simulink library "InverterLIB"  (R2019a)
settings: Solver=VariableStepAuto  StartTime=0.0  StopTime=10.0  RelTol=1e-3
undefined symbols (not defined in the file or in its folder): fsw, Pmax, PolePairs, Tmax, Ts, Tsc, Vnom
libraries: fl_lib x17, nesl_utility x16, ee_lib x10, eePmsmFieldOrientedControl x2
settings Model: Creator=plewi  LastModifiedBy=plewi

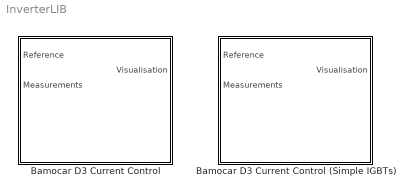
== system InverterLIB ==
  Bamocar D3 Current Control : Subsystem  mask(Bamocar D3){Vnom=Vnom, Pmax=Pmax, Tmax=Tmax, Iq_max=80, p=PolePairs, Vdc_on=10, Ts=2e-6, Tsc=5e-5, c=320, c_unit=uF, Vf=1.45, Ron=1e-3, Goff=1e-5, Vth=0.5, diode_Vf=1.55, diode_Ron=0.001, diode_Goff=1e-5, RefType=Zero d-axis control, psim=0.04, AxisAlignment=Q-axis, Kp_id=0.6, Ki_id=6, Kaw_id=100, Kp_iq=0.2, Ki_iq=8, Kaw_iq=100, AxisPrio=Q-axis, CPWMMode=SVM: space vector modulation, SamplingMode=Natural, fsw=2e3}
      mask prompts: Vnom "Nominal dc-link voltage (V):"; Pmax "Maximum power (W):"; Tmax "Maximum torque (N*m):"; Iq_max "Maximum current, Iq (A):"; p "Number of rotor pole pairs:"; Vdc_on "Inverter dc-link voltage threshold (V):"; Ts "Fundamental sample time (s):"; Tsc "Control sample time (s):"; c "Bank Capacitance"; Vf "Forward voltage, Vf (V):"; Ron "On-state resistance (Ohm):"; Goff "Off-state conductance (Siemens):"; Vth "Threshold voltage, Vth (V):"; diode_Vf "Forward voltage (V):"; diode_Ron "On resistance (Ohm):"; diode_Goff "Off conductance (Siemens):"; RefType "Current references:"; psim "Permanent magnet flux linkage (Wb):"; AxisAlignment "Phase-a axis alignment:"; Kp_id "D-axis current proportional gain:"; Ki_id "D-axis current integral gain:"; Kaw_id "D-axis current anti-windup gain:"; Kp_iq "Q-axis current proportional gain:"; Ki_iq "Q-axis current integral gain:"; Kaw_iq "Q-axis current anti-windup gain:"; AxisPrio "Axis prioritization:"; CPWMMode "PWM method:"; SamplingMode "Sampling mode:"; fsw "Switching frequency (Hz):"
      mask help: This block implements a PMSM field-oriented control structure, similar to the Bamocar D3. It operates under current/torque control.
      mask Help: web(nesl_help(gcbh))
      mask TypeOptions Vnom:
      | Inverter Controller/PMSM Field-Oriented
      | Control/Vnom
      mask TypeOptions Pmax:
      | Inverter Controller/PMSM Field-Oriented
      | Control/Pmax
      mask TypeOptions Tmax:
      | Inverter Controller/PMSM Field-Oriented
      | Control/Tmax
      mask TypeOptions p:
      | Inverter Controller/PMSM Field-Oriented
      | Control/p
      mask TypeOptions Vdc_on:
      | Inverter Controller/PMSM Field-Oriented
      | Control/Vdc_on
      mask TypeOptions Ts:
      | Inverter Controller/PMSM Field-Oriented
      | Control/Ts
      mask TypeOptions Tsc:
      | Inverter Controller/PMSM Field-Oriented
      | Control/Tsc
      mask TypeOptions c:
      | Three-Phase
      | Inverter/Capacitor
      | Bank/c
      mask TypeOptions c_unit:
      | Three-Phase
      | Inverter/Capacitor
      | Bank/c_unit
      mask TypeOptions Vf:
      | Three-Phase
      | Inverter/IGBT A(H)/Vf | Three-Phase
      | Inverter/IGBT A(L)/Vf | Three-Phase
      | Inverter/IGBT B(H)/Vf | Three-Phase
      | Inverter/IGBT B(L)/Vf | Three-Phase
      | Inverter/IGBT C(H)/Vf | Three-Phase
      | Inverter/IGBT C(L)/Vf
      mask TypeOptions Ron:
      | Three-Phase
      | Inverter/IGBT A(H)/Ron | Three-Phase
      | Inverter/IGBT A(L)/Ron | Three-Phase
      | Inverter/IGBT B(H)/Ron | Three-Phase
      | Inverter/IGBT B(L)/Ron | Three-Phase
      | Inverter/IGBT C(H)/Ron | Three-Phase
      | Inverter/IGBT C(L)/Ron
      mask TypeOptions Goff:
      | Three-Phase
      | Inverter/IGBT A(H)/Goff | Three-Phase
      | Inverter/IGBT A(L)/Goff | Three-Phase
      | Inverter/IGBT B(H)/Goff | Three-Phase
      | Inverter/IGBT B(L)/Goff | Three-Phase
      | Inverter/IGBT C(H)/Goff | Three-Phase
      | Inverter/IGBT C(L)/Goff
      mask TypeOptions Vth:
      | Three-Phase
      | Inverter/IGBT A(H)/Vth | Three-Phase
      | Inverter/IGBT A(L)/Vth | Three-Phase
      | Inverter/IGBT B(H)/Vth | Three-Phase
      | Inverter/IGBT B(L)/Vth | Three-Phase
      | Inverter/IGBT C(H)/Vth | Three-Phase
      | Inverter/IGBT C(L)/Vth
      mask TypeOptions diode_Vf:
      | Three-Phase
      | Inverter/IGBT A(H)/diode_Vf | Three-Phase
      | Inverter/IGBT A(L)/diode_Vf | Three-Phase
      | Inverter/IGBT B(H)/diode_Vf | Three-Phase
      | Inverter/IGBT B(L)/diode_Vf | Three-Phase
      | Inverter/IGBT C(H)/diode_Vf | Three-Phase
      | Inverter/IGBT C(L)/diode_Vf
      mask TypeOptions diode_Ron:
      | Three-Phase
      | Inverter/IGBT A(H)/diode_Ron | Three-Phase
      | Inverter/IGBT A(L)/diode_Ron | Three-Phase
      | Inverter/IGBT B(H)/diode_Ron | Three-Phase
      | Inverter/IGBT B(L)/diode_Ron | Three-Phase
      | Inverter/IGBT C(H)/diode_Ron | Three-Phase
      | Inverter/IGBT C(L)/diode_Ron
      mask TypeOptions diode_Goff:
      | Three-Phase
      | Inverter/IGBT A(H)/diode_Goff | Three-Phase
      | Inverter/IGBT A(L)/diode_Goff | Three-Phase
      | Inverter/IGBT B(H)/diode_Goff | Three-Phase
      | Inverter/IGBT B(L)/diode_Goff | Three-Phase
      | Inverter/IGBT C(H)/diode_Goff | Three-Phase
      | Inverter/IGBT C(L)/diode_Goff
      mask TypeOptions RefType:
      | Inverter Controller/PMSM Field-Oriented
      | Control/RefType
      mask TypeOptions psim:
      | Inverter Controller/PMSM Field-Oriented
      | Control/psim
      mask TypeOptions AxisAlignment:
      | Inverter Controller/PMSM Field-Oriented
      | Control/AxisAlignment
      mask TypeOptions Kp_id:
      | Inverter Controller/PMSM Field-Oriented
      | Control/Kp_id
      mask TypeOptions Ki_id:
      | Inverter Controller/PMSM Field-Oriented
      | Control/Ki_id
      mask TypeOptions Kaw_id:
      | Inverter Controller/PMSM Field-Oriented
      | Control/Kaw_id
      mask TypeOptions Kp_iq:
      | Inverter Controller/PMSM Field-Oriented
      | Control/Kp_iq
      mask TypeOptions Ki_iq:
      | Inverter Controller/PMSM Field-Oriented
      | Control/Ki_iq
      mask TypeOptions Kaw_iq:
      | Inverter Controller/PMSM Field-Oriented
      | Control/Kaw_iq
      mask TypeOptions AxisPrio:
      | Inverter Controller/PMSM Field-Oriented
      | Control/AxisPrio
      mask TypeOptions CPWMMode:
      | Inverter Controller/PMSM Field-Oriented
      | Control/CPWMMode
      mask TypeOptions SamplingMode:
      | Inverter Controller/PMSM Field-Oriented
      | Control/SamplingMode
      mask TypeOptions fsw:
      | Inverter Controller/PMSM Field-Oriented
      | Control/fsw
      mask DialogControl Container4 Prompt: General
      mask DialogControl Container11 Prompt: Electrical
      mask DialogControl Container12 Prompt: Capacitor Bank
      mask DialogControl Container16 Prompt: IGBTs
      mask DialogControl Container17 Prompt: Protection Diodes
      mask DialogControl Container5 Prompt: Outer Loop
      mask DialogControl Container6 Prompt: Inner Loop
      mask DialogControl Container7 Prompt: PWM
      mask Display: image('C:\Users\plewi\Documents\University\6-Sixth Year\MUR\MUR-E_Simulation_2019\Images\bamocar_d3.PNG');
  Bamocar D3 Current Control (Simple IGBTs) : Subsystem  mask(Bamocar D3 Current Controlled (Simple Diode)){Vnom=Vnom, Pmax=Pmax, Tmax=Tmax, Iq_max=80, p=PolePairs, Vdc_on=10, Ts=Ts, Tsc=Tsc, Ron=0.01, Goff=1e-8, Vf=0, diode_Vf=1.55, diode_Ron=0.01, diode_Goff=1e-8, RefType=Zero d-axis control, psim=0.04, AxisAlignment=Q-axis, Kp_id=0.6, Ki_id=6, Kaw_id=100, Kp_iq=0.2, Ki_iq=8, Kaw_iq=100, AxisPrio=Q-axis, CPWMMode=SVM: space vector modulation, SamplingMode=Natural, fsw=fsw}
      mask prompts: Vnom "Nominal dc-link voltage (V):"; Pmax "Maximum power (W):"; Tmax "Maximum torque (N*m):"; Iq_max "Maximum current, Iq (A):"; p "Number of rotor pole pairs:"; Vdc_on "Inverter dc-link voltage threshold (V):"; Ts "Fundamental sample time (s):"; Tsc "Control sample time (s):"; Ron "On-state resistance (Ohm):"; Goff "Off-state conductance (Siemens):"; Vf "Switching Threshold:"; diode_Vf "Forward voltage (V):"; diode_Ron "On resistance (Ohm):"; diode_Goff "Off conductance (Siemens):"; RefType "Current references:"; psim "Permanent magnet flux linkage (Wb):"; AxisAlignment "Phase-a axis alignment:"; Kp_id "D-axis current proportional gain:"; Ki_id "D-axis current integral gain:"; Kaw_id "D-axis current anti-windup gain:"; Kp_iq "Q-axis current proportional gain:"; Ki_iq "Q-axis current integral gain:"; Kaw_iq "Q-axis current anti-windup gain:"; AxisPrio "Axis prioritization:"; CPWMMode "PWM method:"; SamplingMode "Sampling mode:"; fsw "Switching frequency (Hz):"
      mask help: This block implements a PMSM field-oriented control structure, similar to the Bamocar D3. It operates under current/torque control.
      mask Help: web(nesl_help(gcbh))
      mask TypeOptions Vnom:
      | Inverter Controller/PMSM Field-Oriented
      | Control/Vnom
      mask TypeOptions Pmax:
      | Inverter Controller/PMSM Field-Oriented
      | Control/Pmax
      mask TypeOptions Tmax:
      | Inverter Controller/PMSM Field-Oriented
      | Control/Tmax
      mask TypeOptions p:
      | Inverter Controller/PMSM Field-Oriented
      | Control/p
      mask TypeOptions Vdc_on:
      | Inverter Controller/PMSM Field-Oriented
      | Control/Vdc_on
      mask TypeOptions Ts:
      | Inverter Controller/PMSM Field-Oriented
      | Control/Ts
      mask TypeOptions Tsc:
      | Inverter Controller/PMSM Field-Oriented
      | Control/Tsc
      mask TypeOptions Ron:
      | Three-Phase
      | Inverter/Switch/R_closed | Three-Phase
      | Inverter/Switch1/R_closed | Three-Phase
      | Inverter/Switch2/R_closed | Three-Phase
      | Inverter/Switch3/R_closed | Three-Phase
      | Inverter/Switch4/R_closed | Three-Phase
      | Inverter/Switch5/R_closed
      mask TypeOptions Goff:
      | Three-Phase
      | Inverter/Switch/G_open | Three-Phase
      | Inverter/Switch1/G_open | Three-Phase
      | Inverter/Switch2/G_open | Three-Phase
      | Inverter/Switch3/G_open | Three-Phase
      | Inverter/Switch4/G_open | Three-Phase
      | Inverter/Switch5/G_open
      mask TypeOptions Vf:
      | Three-Phase
      | Inverter/Switch/Threshold | Three-Phase
      | Inverter/Switch1/Threshold | Three-Phase
      | Inverter/Switch2/Threshold | Three-Phase
      | Inverter/Switch3/Threshold | Three-Phase
      | Inverter/Switch4/Threshold | Three-Phase
      | Inverter/Switch5/Threshold
      mask TypeOptions diode_Vf:
      | Three-Phase
      | Inverter/Diode1/Vf | Three-Phase
      | Inverter/Diode2/Vf | Three-Phase
      | Inverter/Diode3/Vf | Three-Phase
      | Inverter/Diode4/Vf | Three-Phase
      | Inverter/Diode5/Vf | Three-Phase
      | Inverter/Diode6/Vf
      mask TypeOptions diode_Ron:
      | Three-Phase
      | Inverter/Diode1/Ron | Three-Phase
      | Inverter/Diode2/Ron | Three-Phase
      | Inverter/Diode3/Ron | Three-Phase
      | Inverter/Diode4/Ron | Three-Phase
      | Inverter/Diode5/Ron | Three-Phase
      | Inverter/Diode6/Ron
      mask TypeOptions diode_Goff:
      | Three-Phase
      | Inverter/Diode1/Goff | Three-Phase
      | Inverter/Diode2/Goff | Three-Phase
      | Inverter/Diode3/Goff | Three-Phase
      | Inverter/Diode4/Goff | Three-Phase
      | Inverter/Diode5/Goff | Three-Phase
      | Inverter/Diode6/Goff
      mask TypeOptions RefType:
      | Inverter Controller/PMSM Field-Oriented
      | Control/RefType
      mask TypeOptions psim:
      | Inverter Controller/PMSM Field-Oriented
      | Control/psim
      mask TypeOptions AxisAlignment:
      | Inverter Controller/PMSM Field-Oriented
      | Control/AxisAlignment
      mask TypeOptions Kp_id:
      | Inverter Controller/PMSM Field-Oriented
      | Control/Kp_id
      mask TypeOptions Ki_id:
      | Inverter Controller/PMSM Field-Oriented
      | Control/Ki_id
      mask TypeOptions Kaw_id:
      | Inverter Controller/PMSM Field-Oriented
      | Control/Kaw_id
      mask TypeOptions Kp_iq:
      | Inverter Controller/PMSM Field-Oriented
      | Control/Kp_iq
      mask TypeOptions Ki_iq:
      | Inverter Controller/PMSM Field-Oriented
      | Control/Ki_iq
      mask TypeOptions Kaw_iq:
      | Inverter Controller/PMSM Field-Oriented
      | Control/Kaw_iq
      mask TypeOptions AxisPrio:
      | Inverter Controller/PMSM Field-Oriented
      | Control/AxisPrio
      mask TypeOptions CPWMMode:
      | Inverter Controller/PMSM Field-Oriented
      | Control/CPWMMode
      mask TypeOptions SamplingMode:
      | Inverter Controller/PMSM Field-Oriented
      | Control/SamplingMode
      mask TypeOptions fsw:
      | Inverter Controller/PMSM Field-Oriented
      | Control/fsw
      mask DialogControl Container4 Prompt: General
      mask DialogControl Container11 Prompt: Electrical
      mask DialogControl Container12 Prompt: Capacitor Bank
      mask DialogControl Container16 Prompt: IGBTs
      mask DialogControl Container17 Prompt: Protection Diodes
      mask DialogControl Container5 Prompt: Outer Loop
      mask DialogControl Container6 Prompt: Inner Loop
      mask DialogControl Container7 Prompt: PWM
      mask Display: image('C:\Users\plewi\Documents\University\6-Sixth Year\MUR\MUR-E_Simulation_2019\Images\bamocar_d3.PNG');

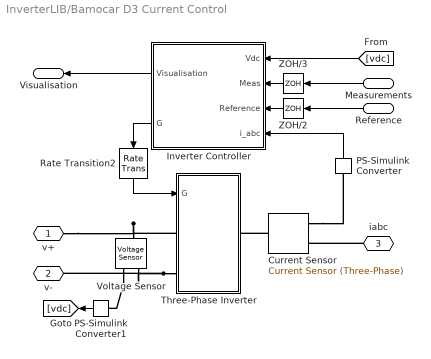
== system InverterLIB/Bamocar D3 Current Control ==
  Reference : Inport
  Measurements : Inport  Port=2
  Current Sensor : ee_lib/Sensors & Transducers/Current Sensor (Three-Phase)
      settings: SourceProductName=Simscape Electrical
  Inverter Controller : Subsystem
  PS-Simulink Converter : nesl_utility/PS-Simulink Converter  PhysicalDomain=network_engine_domain  SubClassName=ps_output  LeftPortType=input  RightPortType=output  PseudoPeriodic=off  Frequencies=[]  Unit=1  AffineConversion=off
  PS-Simulink Converter1 : nesl_utility/PS-Simulink Converter  PhysicalDomain=network_engine_domain  SubClassName=ps_output  LeftPortType=input  RightPortType=output  PseudoPeriodic=off  Frequencies=[]  Unit=1  AffineConversion=off
  Rate Transition2 : RateTransition  OutPortSampleTime=Ts
  Three-Phase Inverter : Subsystem
  Voltage Sensor : fl_lib/Electrical/Electrical Sensors/Voltage Sensor
  ZOH/2 : ZeroOrderHold  SampleTime=Tsc
  ZOH/3 : ZeroOrderHold  SampleTime=Tsc
  v+ : PMIOPort  Side=Left
  v- : PMIOPort  Port=2  Side=Left
  iabc : PMIOPort  Port=3  Side=Right
  Visualisation : Outport
  wires:
  PS-Simulink Converter/1 -> Inverter Controller/4(i_abc)
  ZOH/2/1 -> Inverter Controller/3(Reference)
  Rate Transition2/1 -> Three-Phase Inverter/1(G)
  Measurements/1 -> ZOH/3/1
  Inverter Controller/1(Visualisation) -> Visualisation/1
  PS-Simulink Converter1/1 -> [vdc]
  Inverter Controller/2(G) -> Rate Transition2/1
  [vdc] -> Inverter Controller/1(Vdc)
  ZOH/3/1 -> Inverter Controller/2(Meas)
  Reference/1 -> ZOH/2/1
  connections:
  Voltage Sensor/LConn1 -- v+/RConn1 -- Three-Phase Inverter/LConn1
  Three-Phase Inverter/LConn2 -- v-/RConn1 -- Voltage Sensor/RConn2
  Current Sensor/LConn1 -- Three-Phase Inverter/RConn1
  Current Sensor/RConn1 -- PS-Simulink Converter/LConn1
  Voltage Sensor/RConn1 -- PS-Simulink Converter1/LConn1
  iabc/RConn1 -- Current Sensor/RConn2

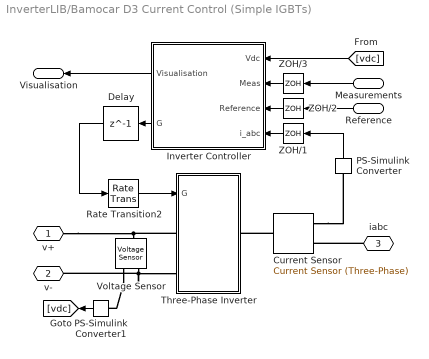
== system InverterLIB/Bamocar D3 Current Control (Simple IGBTs) ==
  Reference : Inport
  Measurements : Inport  Port=2
  Current Sensor : ee_lib/Sensors & Transducers/Current Sensor (Three-Phase)
      settings: SourceProductName=Simscape Electrical
  Delay : Delay  DelayLength=1
  Inverter Controller : Subsystem
  PS-Simulink Converter : nesl_utility/PS-Simulink Converter  PhysicalDomain=network_engine_domain  SubClassName=ps_output  LeftPortType=input  RightPortType=output  PseudoPeriodic=off  Frequencies=[]  Unit=1  AffineConversion=off
  PS-Simulink Converter1 : nesl_utility/PS-Simulink Converter  PhysicalDomain=network_engine_domain  SubClassName=ps_output  LeftPortType=input  RightPortType=output  PseudoPeriodic=off  Frequencies=[]  Unit=1  AffineConversion=off
  Rate Transition2 : RateTransition  OutPortSampleTime=Ts
  Three-Phase Inverter : Subsystem
  Voltage Sensor : fl_lib/Electrical/Electrical Sensors/Voltage Sensor
  ZOH/1 : ZeroOrderHold  SampleTime=Tsc
  ZOH/2 : ZeroOrderHold  SampleTime=Tsc
  ZOH/3 : ZeroOrderHold  SampleTime=Tsc
  v+ : PMIOPort  Side=Left
  v- : PMIOPort  Port=2  Side=Left
  iabc : PMIOPort  Port=3  Side=Right
  Visualisation : Outport
  wires:
  Reference/1 -> ZOH/2/1
  ZOH/3/1 -> Inverter Controller/2(Meas)
  [vdc] -> Inverter Controller/1(Vdc)
  PS-Simulink Converter1/1 -> [vdc]
  Inverter Controller/1(Visualisation) -> Visualisation/1
  Rate Transition2/1 -> Three-Phase Inverter/1(G)
  ZOH/2/1 -> Inverter Controller/3(Reference)
  PS-Simulink Converter/1 -> ZOH/1/1
  ZOH/1/1 -> Inverter Controller/4(i_abc)
  Inverter Controller/2(G) -> Delay/1
  Delay/1 -> Rate Transition2/1
  Measurements/1 -> ZOH/3/1
  connections:
  iabc/RConn1 -- Current Sensor/RConn2
  Voltage Sensor/RConn1 -- PS-Simulink Converter1/LConn1
  Current Sensor/RConn1 -- PS-Simulink Converter/LConn1
  Current Sensor/LConn1 -- Three-Phase Inverter/RConn1
  Voltage Sensor/RConn2 -- v-/RConn1 -- Three-Phase Inverter/LConn2
  Three-Phase Inverter/LConn1 -- v+/RConn1 -- Voltage Sensor/LConn1

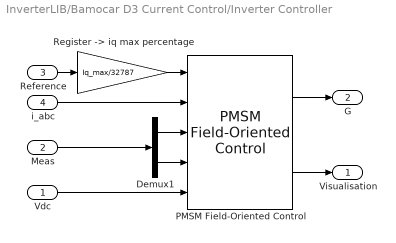
== system InverterLIB/Bamocar D3 Current Control/Inverter Controller ==
  Vdc : Inport
  Meas : Inport  Port=2
  Reference : Inport  Port=3
  i_abc : Inport  Port=4
  Demux1 : Demux  Outputs=2
  PMSM Field-Oriented Control : eePmsmFieldOrientedControl/PMSM Field-Oriented Control  CtrlMode=Torque control  Vnom=Vnom  Pmax=Pmax  Tmax=Tmax  p=p  Vdc_on=Vdc_on  Ts=Ts  Tsc=Tsc  CtrlType=PI control  Kp_w=50  Ki_w=500  Kv_w=1  Kaw_w=1000  RefType=Zero d-axis control  rpmVec=[0, 3000]  TqVec=[-100, 0, 100]  VdcVec=[300, 350]  idMatrix=zeros(2,3,2)  iqMatrix=zeros(2,3,2)  psim=psim  Ld=0.00024  Lq=0.00029  Rs=0.01  AxisAlignment=Q-axis  Kp_id=Kp_id  Ki_id=Ki_id  Kaw_id=Kaw_id  Kp_iq=Kp_iq  Ki_iq=Ki_iq  Kaw_iq=Kaw_iq  AxisPrio=Q-axis  ActZC=on  ActFF=off  ParamTypeFF=Constant parameters  LdFF=Ld  LqFF=Lq  psimFF=PM  idVect=[-200, 0, 200]  iqVect=[-200, 0, 200]  LdMatrix=0.0002 * ones(3, 3)  LqMatrix=0.0002 * ones(3, 3)  psimMatrix=0.04 * ones(3, 3)  CPWMMode=SVM: space vector modulation  fsw=fsw
      settings: SourceProductName=Simscape Electrical  SourceProductBaseCode=PS
  "Register -> iq max percentage" : Gain  Gain=Iq_max/32787
  Visualisation : Outport
  G : Outport  Port=2
  wires:
  PMSM Field-Oriented Control/1 -> G/1
  Vdc/1 -> PMSM Field-Oriented Control/5
  PMSM Field-Oriented Control/2 -> Visualisation/1
  i_abc/1 -> PMSM Field-Oriented Control/2
  Meas/1 -> Demux1/1
  Demux1/1 -> PMSM Field-Oriented Control/3
  Demux1/2 -> PMSM Field-Oriented Control/4
  "Register -> iq max percentage"/1 -> PMSM Field-Oriented Control/1
  Reference/1 -> "Register -> iq max percentage"/1

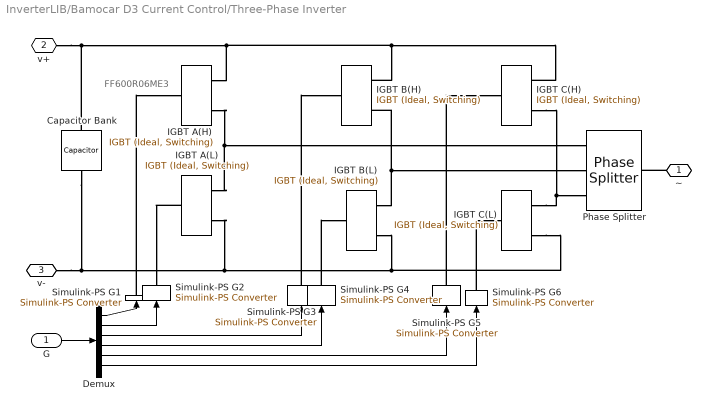
== system InverterLIB/Bamocar D3 Current Control/Three-Phase Inverter ==
  note: FF600R06ME3
  G : Inport
  Capacitor Bank : fl_lib/Electrical/Electrical Elements/Capacitor  c=c uF  r=0 Ohm  g=0 1/Ohm  i_specify=off  i_priority=None  i=0 A  i_nominal_specify=off  i_nominal_unit=A  i_nominal_value=1  v_specify=off  v_priority=None  v=0 V  v_nominal_specify=off  v_nominal_unit=V  v_nominal_value=1  vc_specify=off  vc_priority=High  vc=0 V  vc_nominal_specify=off  vc_nominal_unit=V  vc_nominal_value=1
  Demux : Demux  Outputs=6
  IGBT A(H) : ee_lib/Semiconductors & Converters/IGBT (Ideal, Switching)  Description=Bamocar D3 IGBT Model Number: FF600R06ME3  Vf=Vf V  Ron=Ron Ohm  Goff=Goff S  Vth=Vth V  diode_param=2  diode_Vf=diode_Vf V  diode_Ron=diode_Ron Ohm  diode_Goff=diode_Goff S  diode_C=5e-8 F  diode_iRM=-235 A  diode_iF=300 A  diode_idot=-50 A/us  diode_trr_param=1  diode_trr_factor=3  diode_trr=15 us  diode_Qrr=1.5e+3 s*uA  thermal_loss_option=2  Voff=300 V  Tau=1e-4 s  Tj=[298.15, 398.15] K  Iout_scalar=600 A  Eon_scalar=22.86e-3 J  Eoff_scalar=17.14e-3 J  Von_scalar=2.7 V  Iout_data=[0, 10, 50, 100, 200, 400, 600] A  Eon_data=[0, .29, 1.43, 2.86, 5.71, 13.14, 22.86; 0, .57, 2.63, 5.14, 10.29, 20.57, 30.29] * 1e-3 J  Eoff_data=[0, .21, 1.07, 2.14, 4.29, 9.86, 17.14; 0, .43, 1.97, 3.86, 7.71, 15.43, 22.71] * 1e-3 J  Von_data=[0, 1.1, 1.3, 1.45, 1.75, 2.25, 2.7; 0, 1, 1.15, 1.35, 1.7, 2.35, 3] V
      settings: SourceProductName=Simscape Electrical
  IGBT A(L) : ee_lib/Semiconductors & Converters/IGBT (Ideal, Switching)  Description=Bamocar D3 IGBT Model Number: FF600R06ME3  Vf=Vf V  Ron=Ron Ohm  Goff=Goff S  Vth=Vth V  diode_param=2  diode_Vf=diode_Vf V  diode_Ron=diode_Ron Ohm  diode_Goff=diode_Goff S  diode_C=5e-8 F  diode_iRM=-235 A  diode_iF=300 A  diode_idot=-50 A/us  diode_trr_param=1  diode_trr_factor=3  diode_trr=15 us  diode_Qrr=1.5e+3 s*uA  thermal_loss_option=2  Voff=300 V  Tau=1e-4 s  Tj=[298.15, 398.15] K  Iout_scalar=600 A  Eon_scalar=22.86e-3 J  Eoff_scalar=17.14e-3 J  Von_scalar=2.7 V  Iout_data=[0, 10, 50, 100, 200, 400, 600] A  Eon_data=[0, .29, 1.43, 2.86, 5.71, 13.14, 22.86; 0, .57, 2.63, 5.14, 10.29, 20.57, 30.29] * 1e-3 J  Eoff_data=[0, .21, 1.07, 2.14, 4.29, 9.86, 17.14; 0, .43, 1.97, 3.86, 7.71, 15.43, 22.71] * 1e-3 J  Von_data=[0, 1.1, 1.3, 1.45, 1.75, 2.25, 2.7; 0, 1, 1.15, 1.35, 1.7, 2.35, 3] V
      settings: SourceProductName=Simscape Electrical
  IGBT B(H) : ee_lib/Semiconductors & Converters/IGBT (Ideal, Switching)  Description=Bamocar D3 IGBT Model Number: FF600R06ME3  Vf=Vf V  Ron=Ron Ohm  Goff=Goff S  Vth=Vth V  diode_param=2  diode_Vf=diode_Vf V  diode_Ron=diode_Ron Ohm  diode_Goff=diode_Goff S  diode_C=5e-8 F  diode_iRM=-235 A  diode_iF=300 A  diode_idot=-50 A/us  diode_trr_param=1  diode_trr_factor=3  diode_trr=15 us  diode_Qrr=1.5e+3 s*uA  thermal_loss_option=2  Voff=300 V  Tau=1e-4 s  Tj=[298.15, 398.15] K  Iout_scalar=600 A  Eon_scalar=22.86e-3 J  Eoff_scalar=17.14e-3 J  Von_scalar=2.7 V  Iout_data=[0, 10, 50, 100, 200, 400, 600] A  Eon_data=[0, .29, 1.43, 2.86, 5.71, 13.14, 22.86; 0, .57, 2.63, 5.14, 10.29, 20.57, 30.29] * 1e-3 J  Eoff_data=[0, .21, 1.07, 2.14, 4.29, 9.86, 17.14; 0, .43, 1.97, 3.86, 7.71, 15.43, 22.71] * 1e-3 J  Von_data=[0, 1.1, 1.3, 1.45, 1.75, 2.25, 2.7; 0, 1, 1.15, 1.35, 1.7, 2.35, 3] V
      settings: SourceProductName=Simscape Electrical
  IGBT B(L) : ee_lib/Semiconductors & Converters/IGBT (Ideal, Switching)  Description=Bamocar D3 IGBT Model Number: FF600R06ME3  Vf=Vf V  Ron=Ron Ohm  Goff=Goff S  Vth=Vth V  diode_param=2  diode_Vf=diode_Vf V  diode_Ron=diode_Ron Ohm  diode_Goff=diode_Goff S  diode_C=5e-8 F  diode_iRM=-235 A  diode_iF=300 A  diode_idot=-50 A/us  diode_trr_param=1  diode_trr_factor=3  diode_trr=15 us  diode_Qrr=1.5e+3 s*uA  thermal_loss_option=2  Voff=300 V  Tau=1e-4 s  Tj=[298.15, 398.15] K  Iout_scalar=600 A  Eon_scalar=22.86e-3 J  Eoff_scalar=17.14e-3 J  Von_scalar=2.7 V  Iout_data=[0, 10, 50, 100, 200, 400, 600] A  Eon_data=[0, .29, 1.43, 2.86, 5.71, 13.14, 22.86; 0, .57, 2.63, 5.14, 10.29, 20.57, 30.29] * 1e-3 J  Eoff_data=[0, .21, 1.07, 2.14, 4.29, 9.86, 17.14; 0, .43, 1.97, 3.86, 7.71, 15.43, 22.71] * 1e-3 J  Von_data=[0, 1.1, 1.3, 1.45, 1.75, 2.25, 2.7; 0, 1, 1.15, 1.35, 1.7, 2.35, 3] V
      settings: SourceProductName=Simscape Electrical
  IGBT C(H) : ee_lib/Semiconductors & Converters/IGBT (Ideal, Switching)  Description=Bamocar D3 IGBT Model Number: FF600R06ME3  Vf=Vf V  Ron=Ron Ohm  Goff=Goff S  Vth=Vth V  diode_param=2  diode_Vf=diode_Vf V  diode_Ron=diode_Ron Ohm  diode_Goff=diode_Goff S  diode_C=5e-8 F  diode_iRM=-235 A  diode_iF=300 A  diode_idot=-50 A/us  diode_trr_param=1  diode_trr_factor=3  diode_trr=15 us  diode_Qrr=1.5e+3 s*uA  thermal_loss_option=2  Voff=300 V  Tau=1e-4 s  Tj=[298.15, 398.15] K  Iout_scalar=600 A  Eon_scalar=22.86e-3 J  Eoff_scalar=17.14e-3 J  Von_scalar=2.7 V  Iout_data=[0, 10, 50, 100, 200, 400, 600] A  Eon_data=[0, .29, 1.43, 2.86, 5.71, 13.14, 22.86; 0, .57, 2.63, 5.14, 10.29, 20.57, 30.29] * 1e-3 J  Eoff_data=[0, .21, 1.07, 2.14, 4.29, 9.86, 17.14; 0, .43, 1.97, 3.86, 7.71, 15.43, 22.71] * 1e-3 J  Von_data=[0, 1.1, 1.3, 1.45, 1.75, 2.25, 2.7; 0, 1, 1.15, 1.35, 1.7, 2.35, 3] V
      settings: SourceProductName=Simscape Electrical
  IGBT C(L) : ee_lib/Semiconductors & Converters/IGBT (Ideal, Switching)  Description=Bamocar D3 IGBT Model Number: FF600R06ME3  Vf=Vf V  Ron=Ron Ohm  Goff=Goff S  Vth=Vth V  diode_param=2  diode_Vf=diode_Vf V  diode_Ron=diode_Ron Ohm  diode_Goff=diode_Goff S  diode_C=5e-8 F  diode_iRM=-235 A  diode_iF=300 A  diode_idot=-50 A/us  diode_trr_param=1  diode_trr_factor=3  diode_trr=15 us  diode_Qrr=1.5e+3 s*uA  thermal_loss_option=2  Voff=300 V  Tau=1e-4 s  Tj=[298.15, 398.15] K  Iout_scalar=600 A  Eon_scalar=22.86e-3 J  Eoff_scalar=17.14e-3 J  Von_scalar=2.7 V  Iout_data=[0, 10, 50, 100, 200, 400, 600] A  Eon_data=[0, .29, 1.43, 2.86, 5.71, 13.14, 22.86; 0, .57, 2.63, 5.14, 10.29, 20.57, 30.29] * 1e-3 J  Eoff_data=[0, .21, 1.07, 2.14, 4.29, 9.86, 17.14; 0, .43, 1.97, 3.86, 7.71, 15.43, 22.71] * 1e-3 J  Von_data=[0, 1.1, 1.3, 1.45, 1.75, 2.25, 2.7; 0, 1, 1.15, 1.35, 1.7, 2.35, 3] V
      settings: SourceProductName=Simscape Electrical
  Phase Splitter : ee_lib/Connectors & References/Phase Splitter
      settings: SourceProductName=Simscape Electrical  SourceProductBaseCode=PS
  Simulink-PS G{1..6} (6 alike) : nesl_utility/Simulink-PS Converter  PhysicalDomain=network_engine_domain  SubClassName=ps_input  LeftPortType=input  RightPortType=output  PseudoPeriodic=off  Frequencies=[]  NoiseDistribution=none  NoiseParameters=[]  Unit=1  AffineConversion=off  FilteringAndDerivatives=zero  SimscapeFilterOrder=1  InputFilterTimeConstant=1e-6  UdotUserProvided=0
  ~ : PMIOPort  Tag=PMCPort  Side=Right
  v+ : PMIOPort  Tag=PMCPort  Port=2  Side=Left
  v- : PMIOPort  Tag=PMCPort  Port=3  Side=Left
  wires:
  Demux/5 -> Simulink-PS G5/1
  Demux/4 -> Simulink-PS G4/1
  Demux/3 -> Simulink-PS G3/1
  Demux/2 -> Simulink-PS G2/1
  Demux/1 -> Simulink-PS G1/1
  G/1 -> Demux/1
  Demux/6 -> Simulink-PS G6/1
  connections:
  Simulink-PS G6/RConn1 -- IGBT C(L)/LConn1
  Simulink-PS G5/RConn1 -- IGBT C(H)/LConn1
  Simulink-PS G4/RConn1 -- IGBT B(L)/LConn1
  Simulink-PS G3/RConn1 -- IGBT B(H)/LConn1
  IGBT B(L)/RConn2 -- v-/RConn1 -- Capacitor Bank/RConn1 -- IGBT A(L)/RConn2 -- IGBT C(L)/RConn2
  IGBT A(H)/RConn2 -- Phase Splitter/RConn1 -- IGBT A(L)/RConn1
  IGBT B(L)/RConn1 -- Phase Splitter/RConn2 -- IGBT B(H)/RConn2
  IGBT C(L)/RConn1 -- Phase Splitter/RConn3 -- IGBT C(H)/RConn2
  IGBT B(H)/RConn1 -- Capacitor Bank/LConn1 -- v+/RConn1 -- IGBT A(H)/RConn1 -- IGBT C(H)/RConn1
  ~/RConn1 -- Phase Splitter/LConn1
  Simulink-PS G1/RConn1 -- IGBT A(H)/LConn1
  IGBT A(L)/LConn1 -- Simulink-PS G2/RConn1

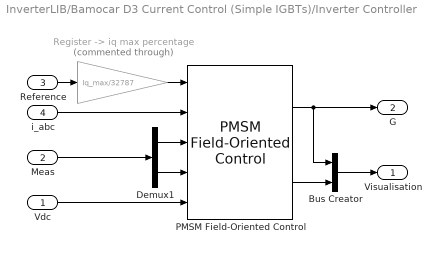
== system InverterLIB/Bamocar D3 Current Control (Simple IGBTs)/Inverter Controller ==
  Vdc : Inport
  Meas : Inport  Port=2
  Reference : Inport  Port=3
  i_abc : Inport  Port=4
  Bus Creator : BusCreator  Inputs=2
  Demux1 : Demux  Outputs=2
  PMSM Field-Oriented Control : eePmsmFieldOrientedControl/PMSM Field-Oriented Control  CtrlMode=Torque control  Vnom=Vnom  Pmax=Pmax  Tmax=Tmax  p=p  Vdc_on=Vdc_on  Ts=Ts  Tsc=Tsc  CtrlType=PI control  Kp_w=50  Ki_w=500  Kv_w=1  Kaw_w=1000  RefType=Zero d-axis control  rpmVec=[0, 3000]  TqVec=[-100, 0, 100]  VdcVec=[300, 350]  idMatrix=zeros(2,3,2)  iqMatrix=zeros(2,3,2)  psim=psim  Ld=0.00024  Lq=0.00029  Rs=0.01  AxisAlignment=Q-axis  Kp_id=Kp_id  Ki_id=Ki_id  Kaw_id=Kaw_id  Kp_iq=Kp_iq  Ki_iq=Ki_iq  Kaw_iq=Kaw_iq  AxisPrio=Q-axis  ActZC=on  ActFF=off  ParamTypeFF=Constant parameters  LdFF=Ld  LqFF=Lq  psimFF=PM  idVect=[-200, 0, 200]  iqVect=[-200, 0, 200]  LdMatrix=0.0002 * ones(3, 3)  LqMatrix=0.0002 * ones(3, 3)  psimMatrix=0.04 * ones(3, 3)  CPWMMode=SVM: space vector modulation  fsw=fsw
      settings: SourceProductName=Simscape Electrical  SourceProductBaseCode=PS
  "Register -> iq max percentage" : Gain  Commented=through  Gain=Iq_max/32787
  Visualisation : Outport
  G : Outport  Port=2
  wires:
  Reference/1 -> "Register -> iq max percentage"/1
  "Register -> iq max percentage"/1 -> PMSM Field-Oriented Control/1
  Demux1/2 -> PMSM Field-Oriented Control/4
  Demux1/1 -> PMSM Field-Oriented Control/3
  Meas/1 -> Demux1/1
  i_abc/1 -> PMSM Field-Oriented Control/2
  Vdc/1 -> PMSM Field-Oriented Control/5
  PMSM Field-Oriented Control/1 -> Bus Creator/1, G/1
  PMSM Field-Oriented Control/2 -> Bus Creator/2
  Bus Creator/1 -> Visualisation/1

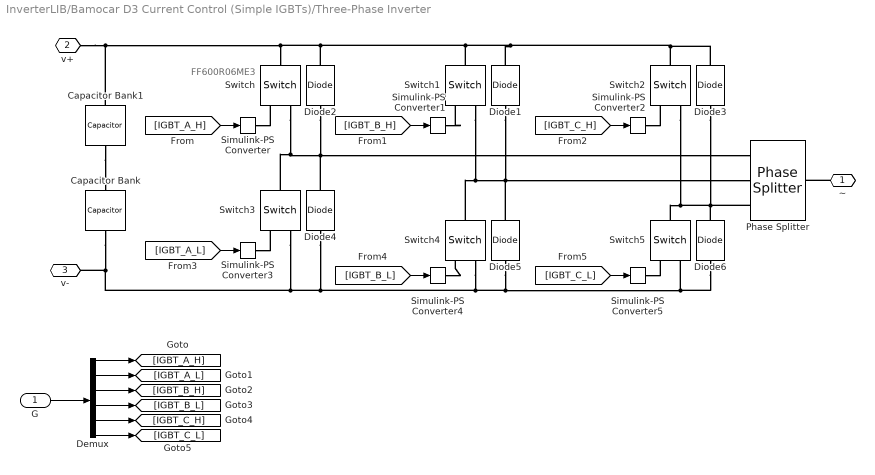
== system InverterLIB/Bamocar D3 Current Control (Simple IGBTs)/Three-Phase Inverter ==
  note: FF600R06ME3
  G : Inport
  Capacitor Bank : fl_lib/Electrical/Electrical Elements/Capacitor  c=320/2 uF  r=0 Ohm  g=0 1/Ohm  i_specify=off  i_priority=None  i=0 A  i_nominal_specify=off  i_nominal_unit=A  i_nominal_value=1  v_specify=off  v_priority=None  v=0 V  v_nominal_specify=off  v_nominal_unit=V  v_nominal_value=1  vc_specify=on  vc_priority=High  vc=Vnom/2 V  vc_nominal_specify=off  vc_nominal_unit=V  vc_nominal_value=1
  Capacitor Bank1 : fl_lib/Electrical/Electrical Elements/Capacitor  c=320/2 uF  r=0 Ohm  g=0 1/Ohm  i_specify=off  i_priority=None  i=0 A  i_nominal_specify=off  i_nominal_unit=A  i_nominal_value=1  v_specify=off  v_priority=None  v=0 V  v_nominal_specify=off  v_nominal_unit=V  v_nominal_value=1  vc_specify=on  vc_priority=High  vc=Vnom/2 V  vc_nominal_specify=off  vc_nominal_unit=V  vc_nominal_value=1
  Demux : Demux  Outputs=6
  Diode{1..6} (6 alike) : fl_lib/Electrical/Electrical Elements/Diode  Vf=diode_Vf V  Ron=diode_Ron Ohm  Goff=diode_Goff 1/Ohm  i_specify=off  i_priority=None  i=0 A  i_nominal_specify=off  i_nominal_unit=A  i_nominal_value=1  v_specify=off  v_priority=None  v=0 V  v_nominal_specify=off  v_nominal_unit=V  v_nominal_value=1
  Phase Splitter : ee_lib/Connectors & References/Phase Splitter
      settings: SourceProductName=Simscape Electrical  SourceProductBaseCode=PS
  Simulink-PS Converter{,1..5} (6 alike) : nesl_utility/Simulink-PS Converter  PhysicalDomain=network_engine_domain  SubClassName=ps_input  LeftPortType=input  RightPortType=output  PseudoPeriodic=off  Frequencies=[]  NoiseDistribution=none  NoiseParameters=[]  Unit=1  AffineConversion=off  FilteringAndDerivatives=provide  SimscapeFilterOrder=1  InputFilterTimeConstant=0.001  UdotUserProvided=0
  Switch{,1..5} (6 alike) : fl_lib/Electrical/Electrical Elements/Switch  R_closed=Ron Ohm  G_open=Goff 1/Ohm  Threshold=Vf  i_specify=off  i_priority=None  i=0 A  i_nominal_specify=off  i_nominal_unit=A  i_nominal_value=1  v_specify=off  v_priority=None  v=0 V  v_nominal_specify=off  v_nominal_unit=V  v_nominal_value=1
      settings: SourceProductName=Simscape
  ~ : PMIOPort  Tag=PMCPort  Side=Right
  v+ : PMIOPort  Tag=PMCPort  Port=2  Side=Left
  v- : PMIOPort  Tag=PMCPort  Port=3  Side=Left
  wires:
  G/1 -> Demux/1
  [IGBT_A_H] -> Simulink-PS Converter/1
  [IGBT_B_H] -> Simulink-PS Converter1/1
  [IGBT_C_H] -> Simulink-PS Converter2/1
  [IGBT_A_L] -> Simulink-PS Converter3/1
  [IGBT_B_L] -> Simulink-PS Converter4/1
  [IGBT_C_L] -> Simulink-PS Converter5/1
  Demux/1 -> [IGBT_A_H]
  Demux/2 -> [IGBT_A_L]
  Demux/3 -> [IGBT_B_H]
  Demux/4 -> [IGBT_B_L]
  Demux/5 -> [IGBT_C_H]
  Demux/6 -> [IGBT_C_L]
  connections:
  ~/RConn1 -- Phase Splitter/LConn1
  Switch/RConn2 -- Switch3/LConn1 -- Diode4/RConn1 -- Diode2/LConn1 -- Phase Splitter/RConn1
  Capacitor Bank/RConn1 -- Switch3/RConn2 -- Diode4/LConn1 -- Diode6/LConn1 -- Switch5/RConn2 -- Diode5/LConn1 -- Switch4/RConn2 -- v-/RConn1
  v+/RConn1 -- Capacitor Bank1/LConn1 -- Diode1/RConn1 -- Switch2/LConn1 -- Diode3/RConn1 -- Switch1/LConn1 -- Diode2/RConn1 -- Switch/LConn1
  Simulink-PS Converter/RConn1 -- Switch/RConn1
  Simulink-PS Converter1/RConn1 -- Switch1/RConn1
  Simulink-PS Converter2/RConn1 -- Switch2/RConn1
  Simulink-PS Converter3/RConn1 -- Switch3/RConn1
  Simulink-PS Converter4/RConn1 -- Switch4/RConn1
  Simulink-PS Converter5/RConn1 -- Switch5/RConn1
  Switch4/LConn1 -- Switch1/RConn2 -- Phase Splitter/RConn2 -- Diode1/LConn1 -- Diode5/RConn1
  Phase Splitter/RConn3 -- Diode3/LConn1 -- Diode6/RConn1 -- Switch2/RConn2 -- Switch5/LConn1
  Capacitor Bank1/RConn1 -- Capacitor Bank/LConn1
